simulink model "phaselock_demo"  (Simulink 6.0)
settings: Solver=ode45  StartTime=0.0  StopTime=1e-4  MaxStep=1/(4*5e6)  RelTol=1e-1
PreLoadFcn:
  | load phaselock_demo
values from neighbouring files (symbols this model uses):
  k0 = 1    [phaselock_demo.mat]
  k1 = 1    [phaselock_demo.mat]    (also in pitchrate_demo.mat = 0.9)
  k2 = 1    [phaselock_demo.mat]    (also in pitchrate_demo.mat = -0.00807)
  k3 = 1    [phaselock_demo.mat]    (also in pitchrate_demo.mat = -0.475)
  k4 = 1    [phaselock_demo.mat]
libraries: simulink_extras x2, dspddes2 x1, srolib x1, commsynccomp2 x1
settings Model: Creator=ksubbara  LastModifiedBy=rlandy  ExtModeTrigMode=oneshot  ExtModeArmWhenConnect=off  BufferReuse=off
settings DataIOCC: LimitDataPoints=off  SaveOutput=off  SaveTime=off  SignalLoggingName=logsOut
settings OptimizationCC: BooleanDataType=off  OptimizeBlockIOStorage=off  BufferReuse=off  LocalBlockOutputs=off  ParameterPooling=off
settings DebuggingCC: CheckExecutionContextPreStartOutputMsg=on  CheckExecutionContextRuntimeOutputMsg=on  SolverPrmCheckMsg=none
settings HardwareCC: TargetUnknown=on
settings ModelReferenceCC: UpdateModelReferenceTargets=IfOutOfDate
settings SFSimCC: SFSimApplyToAllLibs=on  SFSimBuildMode=Incremental

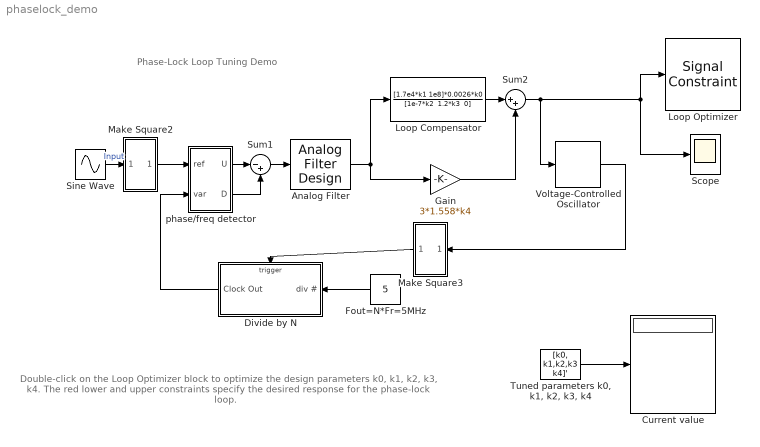
== system phaselock_demo ==
  note: Phase-Lock Loop Tuning Demo
  note: Double-click on the Loop Optimizer block
      | to optimize the design parameters k0, k1, k2, k3, k4.
      |
      | The red lower and upper constraints specify
      | the desired response for the phase-lock loop.
  "Analog Filter " : dspddes2/Analog Filter Design  method=Elliptic  filttype=Lowpass  N=4  Wlo=2*pi*350e3  Whi=80  Rp=3  Rs=80
  Current value : Display
  Divide by N : Subsystem  Orientation=left  AncestorBlock=rab_favorites/Divide by N  TreatAsAtomicUnit=on  PropExecContextAcrossSSBoundary=on
  Fout=N*Fr=5MHz : Constant  Orientation=left  Value=5
  Gain : Gain  Gain=3*1.558*k4  SaturateOnIntegerOverflow=on
  Loop Compensator : TransferFcn  Numerator=[1.7e4*k1 1e8]*0.0026*k0  Denominator="[1e-7*k2  1.2*k3  0]"
  Loop Optimizer : srolib/Signal Constraint  DialogPosition=[0.050625 0.2075 0.38625 0.245]  SaveIn=workspace  SaveAs=OptimProject  LogID=SRO_DataLog_1  Ylim=[-0.5 1.5]
  Make Square2 : Subsystem  PropExecContextAcrossSSBoundary=on
      mask Type: Make Square
      mask Description:
      | For input +ve values output is 1
      | For input -ve values output is 0
      mask Display: plot(0,0,100,100,[90,70,70,50,50,30,30,10,10],[20,20,40,40,20,20,40,40,20],[90,87,84,80,76,73,70,67,63,60,57,53,50,47,44,40,36,33,30,27,23,20,17,13,10],[70,65,63,62,63,65,70,75,77,78,77,75,70,65,63,62,63,65,70,75,77,78,77,75,70])
  Make Square3 : Subsystem  Orientation=left  PropExecContextAcrossSSBoundary=on
      mask Type: Make Square
      mask Description:
      | For input +ve values output is 1
      | For input -ve values output is 0
      mask Display: plot(0,0,100,100,[90,70,70,50,50,30,30,10,10],[20,20,40,40,20,20,40,40,20],[90,87,84,80,76,73,70,67,63,60,57,53,50,47,44,40,36,33,30,27,23,20,17,13,10],[70,65,63,62,63,65,70,75,77,78,77,75,70,65,63,62,63,65,70,75,77,78,77,75,70])
  Scope : Scope
      settings: TimeRange=0.00012  YMin=-0.2  YMax=1.4
  Sine Wave : Sin  Frequency=2*pi*(1e6)  Phase=pi  SampleTime=0
  Sum1 : Sum  Inputs=|-+  SaturateOnIntegerOverflow=on  InputSameDT=on
  Sum2 : Sum  Inputs=|++  SaturateOnIntegerOverflow=on  InputSameDT=on
  "Tuned parameters k0, k1, k2, k3, k4" : Constant  Value=[k0, k1,k2,k3 k4]'  VectorParams1D=off
  Voltage-Controlled Oscillator : commsynccomp2/Voltage-Controlled Oscillator  Ac=1  Fc=4.9e6  Kc=0.1e6  Ph=pi*0.6
  phase/freq detector : Subsystem  PropExecContextAcrossSSBoundary=on
  wires:
  Sine Wave/1 -> Make Square2/1(In1)  "Input"
  Voltage-Controlled Oscillator/1 -> Make Square3/1(In1)
  Make Square2/1(Out1) -> phase/freq detector/1(ref)
  phase/freq detector/1(U) -> Sum1/1
  phase/freq detector/2(D) -> Sum1/2
  Sum1/1 -> "Analog Filter "/1
  Make Square3/1(Out1) -> Divide by N/Trigger
  Fout=N*Fr=5MHz/1 -> Divide by N/1(div #)
  Divide by N/1(Clock Out) -> phase/freq detector/2(var)
  "Tuned parameters k0, k1, k2, k3, k4"/1 -> Current value/1
  Loop Compensator/1 -> Sum2/1
  Gain/1 -> Sum2/2
  Sum2/1 -> Voltage-Controlled Oscillator/1, Loop Optimizer/1, Scope/1
  "Analog Filter "/1 -> Loop Compensator/1, Gain/1

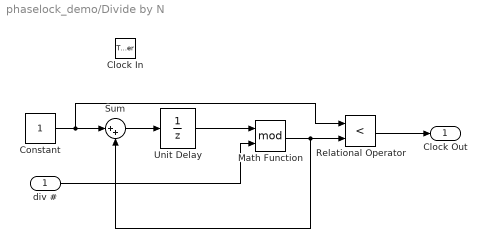
== system phaselock_demo/Divide by N ==
  div # : Inport  LatchInput=off
  Clock In : TriggerPort
  Constant : Constant
  Math Function : Math  Operator=mod  SaturateOnIntegerOverflow=on
  Relational Operator : RelationalOperator  Operator=<  InputSameDT=on
  Sum : Sum  Inputs=|++  SaturateOnIntegerOverflow=on  InputSameDT=on
  Unit Delay : UnitDelay  SampleTime=-1
  Clock Out : Outport
  wires:
  Constant/1 -> Sum/1, Relational Operator/1
  Sum/1 -> Unit Delay/1
  Unit Delay/1 -> Math Function/1
  div #/1 -> Math Function/2
  Math Function/1 -> Sum/2, Relational Operator/2
  Relational Operator/1 -> Clock Out/1

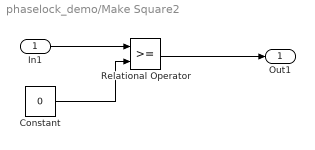
== system phaselock_demo/Make Square2 ==
  In1 : Inport  LatchInput=off
  Constant : Constant  Value=0
  Relational Operator : RelationalOperator  InputSameDT=on
  Out1 : Outport
  wires:
  Relational Operator/1 -> Out1/1
  Constant/1 -> Relational Operator/2
  In1/1 -> Relational Operator/1

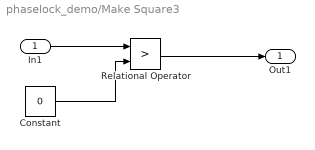
== system phaselock_demo/Make Square3 ==
  In1 : Inport  LatchInput=off
  Constant : Constant  Value=0
  Relational Operator : RelationalOperator  Operator=>  InputSameDT=on
  Out1 : Outport
  wires:
  In1/1 -> Relational Operator/1
  Constant/1 -> Relational Operator/2
  Relational Operator/1 -> Out1/1

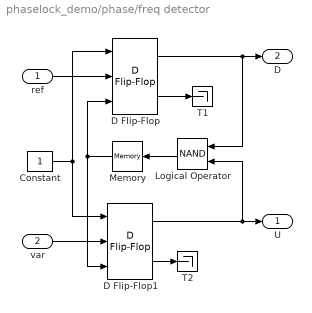
== system phaselock_demo/phase/freq detector ==
  ref : Inport  LatchInput=off
  var : Inport  Port=2  LatchInput=off
  Constant : Constant
  D Flip-Flop : simulink_extras/Flip Flops/D Flip-Flop
  D Flip-Flop1 : simulink_extras/Flip Flops/D Flip-Flop
  Logical Operator : Logic  Orientation=left  Operator=NAND
  Memory : Memory  Orientation=left
  T1 : Terminator
  T2 : Terminator
  U : Outport
  D : Outport  Port=2
  wires:
  ref/1 -> D Flip-Flop/2
  var/1 -> D Flip-Flop1/2
  Constant/1 -> D Flip-Flop/1, D Flip-Flop1/1
  Logical Operator/1 -> Memory/1
  Memory/1 -> D Flip-Flop/3, D Flip-Flop1/3
  D Flip-Flop/1 -> Logical Operator/1, D/1
  D Flip-Flop1/1 -> Logical Operator/2, U/1
  D Flip-Flop/2 -> T1/1
  D Flip-Flop1/2 -> T2/1
